simulink library "librairie_v2006b"  (Simulink 6.5)
values from neighbouring files (symbols this model uses):
  entree_simulink = [t_simulink', code_simulink']    [TP.m]
  fe_simulink = 50000    [TP.m]
  Tsymbole_simulink = 70    [TP.m]
undefined symbols (not defined in the file or in its folder): a, a2, b, b2, in
libraries: simulink x3
settings Model: Creator=sylar  LastModifiedBy=sylar

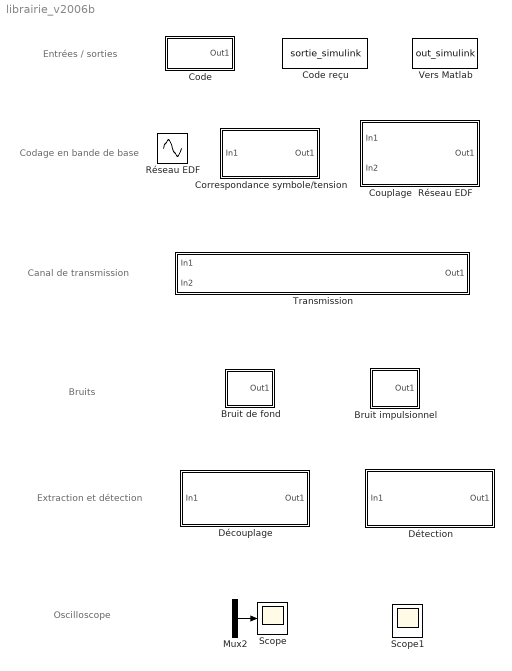
== system librairie_v2006b ==
  note: Entrées / sorties
  note: Codage en
      | bande de base
  note: Canal de
      | transmission
  note: Bruits
  note: Extraction et détection
  note: Oscilloscope
  Bruit de fond : Subsystem  mask{RSB=-5}
      mask prompts: RSB "RSB (dB) ?"
      mask help: Bruit de fond (bruit blanc gaussien)
      mask init:
      | Tsymbole_simulink= evalin('base','Tsymbole_simulink');
      | A_symbole = evalin('base','Asymbole_simulink');
      | x = evalin('base','code');
      | Ex = x*x';
      | 
      | Ey = Tsymbole_simulink*A_symbole^2*(4*Ex - 2*x*ones(length(x),1) - 2*ones(1,length(x))*x' + length(x));
      | Ey = Ey / (length(x) * Tsymbole_simulink);
      mask Display: port_label('output', 1, 'Bruit')
  Bruit impulsionnel : Subsystem  mask{NB=10, AMP=0}
      mask prompts: NB "Nombre d'impulsion"; AMP "Amplitude (V)"
      mask help: Bruit impulsionnel, d'amplitude maximale A.
      mask Display: port_label('output', 1, 'Bruit')
  Code : Subsystem  mask{T_symbole=Tsymbole_simulink}
      mask prompts: T_symbole "Duree d'un symbole"
      mask help: Information (binaire) a transmettre
      mask Display: port_label('output', 1, 'Flux binaire')
  Code reçu : ToWorkspace  VariableName=sortie_simulink  SampleTime=-1  SaveFormat=Array
  Correspondance symbole/tension : Subsystem  mask{A_symbole=5}
      mask prompts: A_symbole "Amplitude d'un symbole"
      mask help: Correspondance symbole binaire / tension
      mask init:
      | assignin('base','A_symbole',A_symbole)
      mask Display:
      | port_label('input', 1, 'Code')
      | port_label('output', 1, 'Tension')
  Couplage  Réseau EDF : Subsystem  mask{fp=10000}
      mask prompts: fp "Frequence porteuse"
      mask help: Couplage de l'information a transmettre sur le reseau EDF
      mask init:
      | assignin('base','fp',fp);
      mask Display:
      | port_label('input', 1, 'Information')
      | port_label('input', 2, 'Secteur')
      | port_label('output', 1, 'Tension')
  Découplage : Subsystem  mask{TOTO=0}
      mask help: Recuperation de l'information superposee au secteur
      mask init:
      | fp = evalin('base','fp');
      | [b,a] = butter(10,2*pi*1000,'high','s');
      | [b2,a2] = butter(10,2*pi*fp/2,'s');
      mask Display:
      | port_label('input', 1, 'Secteur')
      | port_label('output', 1, 'Tension')
  Détection : Subsystem  mask{seuil=0}
      mask prompts: seuil "Valeur du seuil (V)"
      mask help: Detection : la tension correspond-elle a un 0 ou 1 ?
      mask Display:
      | port_label('input', 1, 'Tension')
      | port_label('output', 1, 'Code reçu')
  Mux2 : Mux  Inputs=2
  Réseau EDF : Sin  Amplitude=sqrt(2)*240  Bias=0  Frequency=2*pi*50  Phase=0  Samples=10  SampleTime=0  Offset=0
  Scope : Scope
      settings: YMin=-7  YMax=8
  Scope1 : Scope  NumInputPorts=2
      settings: YMin=0~0  YMax=1~1
  Transmission : Subsystem  mask{TOTO=}
      mask help: Simulation d'un canal de transmission
      mask Display:
      | port_label('input', 1, 'Tension')
      | port_label('input', 2, 'Bruit')
      | port_label('output', 1, 'Secteur')
  Vers Matlab : ToWorkspace  VariableName=out_simulink  SampleTime=1/fe_simulink  SaveFormat=Array
  wires:
  Mux2/1 -> Scope/1

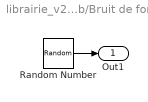
== system librairie_v2006b/Bruit de fond ==
  Random Number : RandomNumber  Variance=Ey/10^(RSB/10)  Seed=fix((rand(1)+1)/2*100)  SampleTime=0
  Out1 : Outport
  wires:
  Random Number/1 -> Out1/1

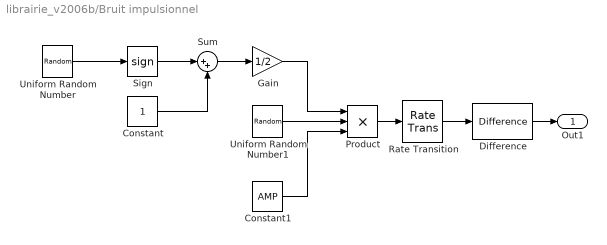
== system librairie_v2006b/Bruit impulsionnel ==
  Constant : Constant  OutDataType=fixdt(1, 16)  OutScaling=2^0
  Constant1 : Constant  Value=AMP  OutDataType=fixdt(1, 16)  OutScaling=2^0
  Difference : simulink/Discrete/Difference  SystemSampleTime=-1  ICPrevInput=0.0  OutDataType=fixdt(1, 16)  OutScaling=2^-10  DoSatur=off
  Gain : Gain  Gain=1/2  ParameterDataType=fixdt(1, 16)  ParameterScaling=2^0  OutDataType=fixdt(1, 16)  OutScaling=2^0
  Product : Product  Inputs=3  OutDataType=fixdt(1, 16)  OutScaling=2^0  SampleTime=fix(length(entree_simulink)/NB)*1/fe_simulink  RndMeth=Zero
  Rate Transition : RateTransition  OutPortSampleTimeMultiple=1/fix(length(in)/5)  OutPortSampleTime=1/fe_simulink/10
  Sign : Signum
  Sum : Sum  Inputs=|++  OutDataType=fixdt(1, 16)  OutScaling=2^0
  Uniform Random Number : UniformRandomNumber  Seed=fix((rand(1)+1)/2*100)  SampleTime=fix(length(entree_simulink)/NB)*1/fe_simulink*Tsymbole_simulink
  Uniform Random Number1 : UniformRandomNumber  Minimum=0  Seed=fix((rand(1)+1)/2*100)  SampleTime=fix(length(entree_simulink)/NB)*1/fe_simulink*Tsymbole_simulink
  Out1 : Outport
  wires:
  Difference/1 -> Out1/1
  Rate Transition/1 -> Difference/1
  Constant1/1 -> Product/3
  Product/1 -> Rate Transition/1
  Uniform Random Number1/1 -> Product/2
  Gain/1 -> Product/1
  Sum/1 -> Gain/1
  Constant/1 -> Sum/2
  Sign/1 -> Sum/1
  Uniform Random Number/1 -> Sign/1

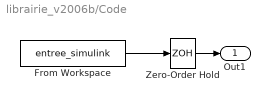
== system librairie_v2006b/Code ==
  From Workspace : FromWorkspace  VariableName=entree_simulink  SampleTime=1/fe_simulink
  Zero-Order Hold : ZeroOrderHold  SampleTime=T_symbole/fe_simulink
  Out1 : Outport
  wires:
  Zero-Order Hold/1 -> Out1/1
  From Workspace/1 -> Zero-Order Hold/1

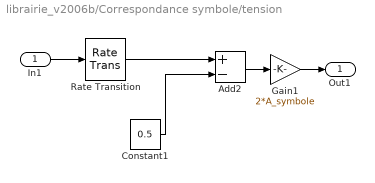
== system librairie_v2006b/Correspondance symbole/tension ==
  In1 : Inport
  Add2 : Sum  Inputs=+-  OutDataType=fixdt(1, 16)  OutScaling=2^-10
  Constant1 : Constant  Value=0.5  OutDataType=fixdt(1, 16)  OutScaling=2^0
  Gain1 : Gain  Gain=2*A_symbole  ParameterDataType=fixdt(1, 16)  ParameterScaling=2^0  OutDataType=fixdt(1, 16)  OutScaling=2^0
  Rate Transition : RateTransition  OutPortSampleTimeMultiple=1/fix(length(in)/5)  OutPortSampleTime=1/fe_simulink
  Out1 : Outport
  wires:
  Gain1/1 -> Out1/1
  In1/1 -> Rate Transition/1
  Rate Transition/1 -> Add2/1
  Add2/1 -> Gain1/1
  Constant1/1 -> Add2/2

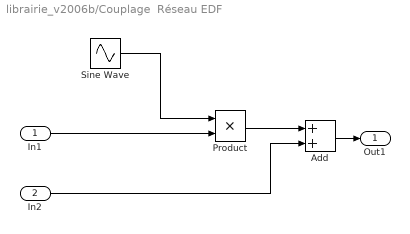
== system librairie_v2006b/Couplage  Réseau EDF ==
  In1 : Inport
  In2 : Inport  Port=2
  Add : Sum  OutDataType=fixdt(1, 16)  OutScaling=2^-10
  Product : Product  OutDataType=fixdt(1, 16)  OutScaling=2^0  RndMeth=Zero
  Sine Wave : Sin  Amplitude=1  Bias=0  Frequency=2*pi*fp  Phase=0  Samples=10  SampleTime=0  Offset=0
  Out1 : Outport
  wires:
  In2/1 -> Add/2
  Add/1 -> Out1/1
  In1/1 -> Product/2
  Product/1 -> Add/1
  Sine Wave/1 -> Product/1

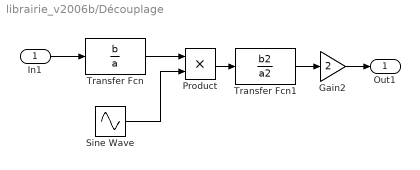
== system librairie_v2006b/Découplage ==
  In1 : Inport
  Gain2 : Gain  Gain=2  ParameterDataType=fixdt(1, 16)  ParameterScaling=2^0  OutDataType=fixdt(1, 16)  OutScaling=2^0
  Product : Product  OutDataType=fixdt(1, 16)  OutScaling=2^0  RndMeth=Zero
  Sine Wave : Sin  Amplitude=1  Bias=0  Frequency=2*pi*fp  Phase=0  Samples=10  SampleTime=0  Offset=0
  Transfer Fcn : TransferFcn  Numerator=b  Denominator=a
  Transfer Fcn1 : TransferFcn  Numerator=b2  Denominator=a2
  Out1 : Outport
  wires:
  Gain2/1 -> Out1/1
  In1/1 -> Transfer Fcn/1
  Transfer Fcn1/1 -> Gain2/1
  Product/1 -> Transfer Fcn1/1
  Sine Wave/1 -> Product/2
  Transfer Fcn/1 -> Product/1

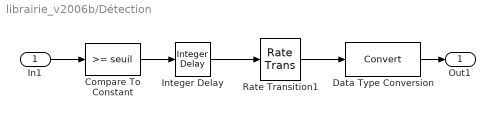
== system librairie_v2006b/Détection ==
  In1 : Inport
  Compare To Constant : simulink/Logic and Bit Operations/Compare To Constant  SystemSampleTime=-1  relop=>=  const=seuil  LogicOutDataTypeMode=boolean
  Data Type Conversion : DataTypeConversion  OutDataTypeMode=double  OutDataType=fixdt(1, 16)  OutScaling=2^0
  Integer Delay : simulink/Discrete/Integer Delay  vinit=0.0  samptime=1/fe_simulink  NumDelays=Tsymbole_simulink/2
  Rate Transition1 : RateTransition  OutPortSampleTimeMultiple=1/fix(length(in)/5)  OutPortSampleTime=Tsymbole_simulink/fe_simulink
  Out1 : Outport
  wires:
  In1/1 -> Compare To Constant/1
  Integer Delay/1 -> Rate Transition1/1
  Compare To Constant/1 -> Integer Delay/1
  Rate Transition1/1 -> Data Type Conversion/1
  Data Type Conversion/1 -> Out1/1

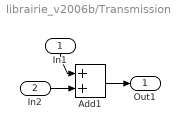
== system librairie_v2006b/Transmission ==
  In1 : Inport  Orientation=down
  In2 : Inport  Port=2
  Add1 : Sum  OutDataType=fixdt(1, 16)  OutScaling=2^-10
  Out1 : Outport
  wires:
  In2/1 -> Add1/2
  Add1/1 -> Out1/1
  In1/1 -> Add1/1
